simulink model "Junctions4Modified"  (Simulink 8.7)
settings: Solver=ode45  StartTime=0.0  StopTime=10.0  RelTol=1e-3
settings Model: Creator=scaife  LastModifiedBy=bourbouh  ExtModeAutoUpdateStatusClock=off
settings DataIOCC: SignalLoggingSaveFormat=ModelDataLogs  SignalLoggingName=sigsOut
settings OptimizationCC: InitFltsAndDblsToZero=on
settings DebuggingCC: SaveWithParameterizedLinksMsg=none  SignalResolutionControl=TryResolveAllWithWarning  MultiTaskDSMMsg=warning  MultiTaskCondExecSysMsg=none  StrictBusMsg=None
settings HardwareCC: TargetUnknown=on
settings SFSimCC: SimParseCustomCode=off
settings GRTTargetCC: TargetFcnLib=ansi_tfl_tmw.mat  ModelReferenceCompliant=off  ParMdlRefBuildCompliant=off  CompOptLevelCompliant=off  ConcurrentExecutionCompliant=off  GeneratePreprocessorConditionals=Use local settings  CombineOutputUpdateFcns=off  MatFileLogging=off  MATLABClassNameForMDSCustomization=Simulink.SoftwareTarget.TargetSpecificTriggerConfigurationBase  GRTInterface=on

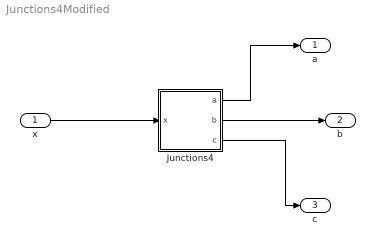
== system Junctions4Modified ==
  x : Inport
  Junctions4 : Stateflow chart  TreatAsAtomicUnit=on
  a : Outport
  b : Outport  Port=2
  c : Outport  Port=3
  wires:
  Junctions4/1(a) -> a/1
  Junctions4/2(b) -> b/1
  Junctions4/3(c) -> c/1
  x/1 -> Junctions4/1(x)

== stateflow chart Junctions4 ==
  state TOP
    state A/
      en:c+=1
      ex:c+=10
    state B/
      en:c+=100
      du:c+=1000
    (default) -> A [order 1] : [x<>0]{a+=10}/b+=10
    (default) -> A [order 2] : [x==0]{a+=1}/b+=1
    A -> (junction 6) [order 2] : [x<4]{a+=100}
    A -> (junction 6) [order 1] : [x>=4]{a+=1000}
    (junction 6) -> B [order 1] : [x%%3<>0]
        | {a+=100000}
        | /b+=100000
    (junction 6) -> B [order 2] : [x%%3==0]
        | {a+=10000}
        | /b+=10000
    B -> TOP
  (default) -> TOP
  data: x input int32; a output int32 =111111; b output int32 =111111; c output int32 =111111
